simulink subsystem "rss_StrtUpRefTqCalcNeed"  (R2023a)
settings: Solver=VariableStepAuto  StartTime=0.0  StopTime=10.0  RelTol=1e-3
undefined symbols (not defined in the file): Cdbl_facStrtUpTqRiseRateMaxVal, Cdbl_nElecAgSpdMaxVal, Cdbl_tiSlwTaskSmpTi, Cdbl_trqTqMaxVal, ENM_MOTO_STATUS, ENM_STRTUP_TRQ_STATUS, Gs16_facStrtUpTqRiseRate_C, Gs16_trqMaxStrtUpTq_C
libraries: simulink x3, lib_conversion x1, lib_discrete_time_integrator x1, vhit_control_library x1
settings Model: Creator=xiaoqiang.yuan  LastModifiedBy=xiaoqiang.yuan

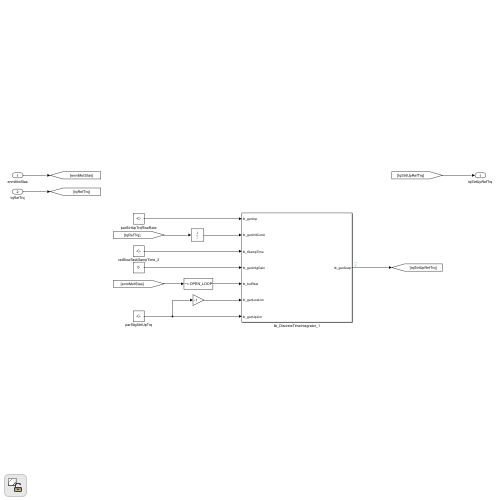
[thumbnail: Simulink's stored preview of the top-level diagram]
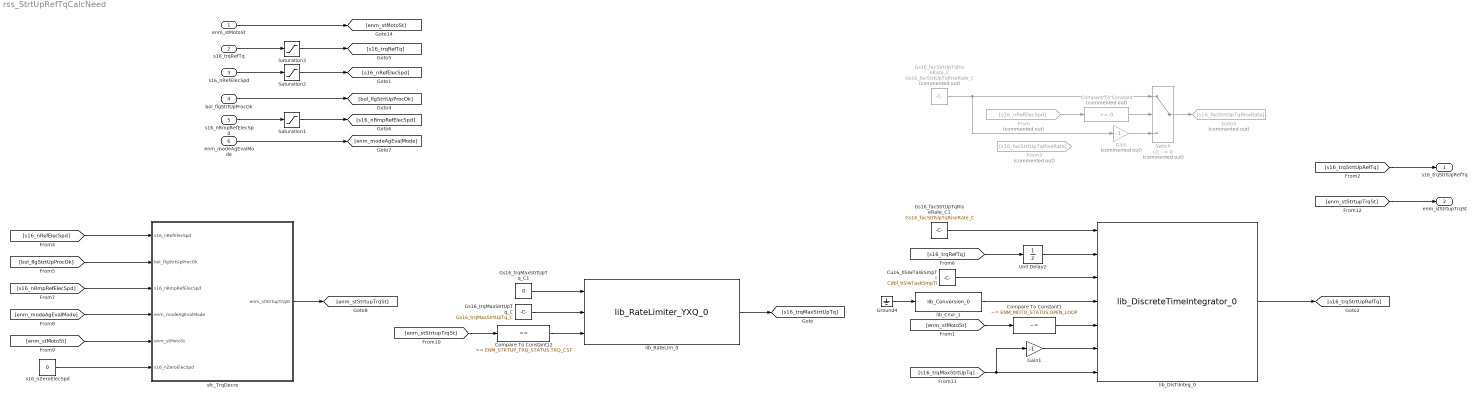
== system rss_StrtUpRefTqCalcNeed ==
  enm_stMotoSt : Inport  OutDataTypeStr=Enum: ENM_MOTO_STATUS
  s16_trqRefTq : Inport  Port=2  OutDataTypeStr=dt_Standardize_s16p15b0
  s16_nRefElecSpd : Inport  Port=3  OutDataTypeStr=dt_Standardize_s16p15b0
  bol_flgStrtUpProcOk : Inport  Port=4  OutDataTypeStr=boolean
  s16_nRmpRefElecSpd : Inport  Port=5  OutDataTypeStr=dt_Standardize_s16p15b0
  enm_modeAgEvalMode : Inport  Port=6  OutDataTypeStr=Enum: ENM_AG_POS_EVAL_MODE
  Compare To Constant : simulink/Logic and Bit Operations/Compare To Constant  Commented=on  relop=>=  const=0  OutDataTypeStr=boolean
  Compare To Constant1 : simulink/Logic and Bit Operations/Compare To Constant  relop=~=  const=ENM_MOTO_STATUS.OPEN_LOOP  OutDataTypeStr=boolean
  Compare To Constant12 : simulink/Logic and Bit Operations/Compare To Constant  relop===  const=ENM_STRTUP_TRQ_STATUS.TRQ_CST  OutDataTypeStr=boolean
  Cu16_tiSlwTaskSmpTi : Constant  Value=Cdbl_tiSlwTaskSmpTi
  From : From  Commented=on  GotoTag=s16_nRefElecSpd
  From3 : From  Commented=on  GotoTag=s16_facStrtUpTqRiseRate
  Gain : Gain  Commented=on  Gain=-1  OutDataTypeStr=Inherit: Same as input
  Gain1 : Gain  Gain=-1  OutDataTypeStr=Inherit: Inherit via back propagation
  Goto3 : Goto  Commented=on  GotoTag=s16_facStrtUpTqRiseRate
  Ground4 : Ground
  Gs16_facStrtUpTqRiseRate_C : Constant  Commented=on  Value=Gs16_facStrtUpTqRiseRate_C  OutDataTypeStr=fixdt(1,16,2^-2,0)
  Gs16_facStrtUpTqRiseRate_C1 : Constant  Value=Gs16_facStrtUpTqRiseRate_C  OutDataTypeStr=fixdt(1,16,2^-2,0)
  Gs16_trqMaxStrtUpTq_C : Constant  Value=Gs16_trqMaxStrtUpTq_C
  Gs16_trqMaxStrtUpTq_C1 : Constant  Value=0  OutDataTypeStr=dt_Standardize_s16p15b0
  Saturation1 : Saturate  UpperLimit=Cdbl_nElecAgSpdMaxVal  LowerLimit=-Cdbl_nElecAgSpdMaxVal
  Saturation2 : Saturate  UpperLimit=Cdbl_nElecAgSpdMaxVal  LowerLimit=-Cdbl_nElecAgSpdMaxVal
  Saturation3 : Saturate  UpperLimit=Cdbl_trqTqMaxVal  LowerLimit=-Cdbl_trqTqMaxVal
  Switch : Switch  Commented=on  Criteria=u2 ~= 0  SaturateOnIntegerOverflow=off  InputSameDT=off
  Unit Delay2 : UnitDelay  SampleTime=-1  HasFrameUpgradeWarning=on
  lib_Cnvr_1 : lib_conversion/lib_Conversion_0  lb_parDataType=uint8  lb_parOutpMaxVal=[]  lb_parOutpMinVal=[]  lb_parSatFlag=off
  lib_DisTiInteg_0 : lib_discrete_time_integrator/lib_DiscreteTimeIntegrator_0  lb_parMaxInpVal=Cdbl_facStrtUpTqRiseRateMaxVal  lb_parMinInpVal=-Cdbl_facStrtUpTqRiseRateMaxVal  lb_parMaxSampTime=double(Cdbl_tiSlwTaskSmpTi)  lb_parMaxIntgGain=0  lb_parAccmDataTypeMode=Same of output  lb_parOutpDataType=dt_Standardize_s16p15b0  lb_parIntgScopMode=Generic signal  lb_parSatFlag=on
  lib_RateLim_0 : vhit_control_library/lib_RateLimiter_YXQ_0  lb_parSampTime=Cdbl_tiSlwTaskSmpTi  lb_parRiseSlewRate=Gs16_facStrtUpTrqDecRiseRate_C  lb_parFallSlewRate=Gs16_facStrtUpTrqDecFallRate_C  lb_parMaxInpVal=Cdbl_trqTqMaxVal  lb_parMinInpVal=-Cdbl_trqTqMaxVal
      settings: LibrarySourceBlock=lib_rate_limiter/lib_RateLimiter_0
  s16_nZeroElecSpd : Constant  Value=0  OutDataTypeStr=dt_Standardize_s16p15b0
  sfc_TrqDecre : Stateflow chart  TreatAsAtomicUnit=on
  s16_trqStrtUpRefTq : Outport  OutDataTypeStr=dt_Standardize_s16p15b0
  enm_stStrtupTrqSt : Outport  Port=2  OutDataTypeStr=Enum: ENM_STRTUP_TRQ_STATUS
  wires:
  Gs16_facStrtUpTqRiseRate_C1/1 -> lib_DisTiInteg_0/1
  [s16_trqStrtUpRefTq] -> s16_trqStrtUpRefTq/1
  lib_Cnvr_1/1 -> lib_DisTiInteg_0/4
  [s16_trqMaxStrtUpTq] -> lib_DisTiInteg_0/7, Gain1/1
  Cu16_tiSlwTaskSmpTi/1 -> lib_DisTiInteg_0/3
  Gain1/1 -> lib_DisTiInteg_0/6
  Compare To Constant1/1 -> lib_DisTiInteg_0/5
  [enm_stMotoSt] -> Compare To Constant1/1
  lib_DisTiInteg_0/1 -> [s16_trqStrtUpRefTq]
  s16_trqRefTq/1 -> Saturation3/1
  [s16_trqRefTq] -> Unit Delay2/1
  Unit Delay2/1 -> lib_DisTiInteg_0/2
  enm_stMotoSt/1 -> [enm_stMotoSt]
  Saturation3/1 -> [s16_trqRefTq]
  Ground4/1 -> lib_Cnvr_1/1
  Saturation2/1 -> [s16_nRefElecSpd]
  s16_nRefElecSpd/1 -> Saturation2/1
  From/1 -> Compare To Constant/1
  Compare To Constant/1 -> Switch/2
  Switch/1 -> Goto3/1
  Gs16_facStrtUpTqRiseRate_C/1 -> Gain/1, Switch/1
  Gain/1 -> Switch/3
  bol_flgStrtUpProcOk/1 -> [bol_flgStrtUpProcOk]
  enm_modeAgEvalMode/1 -> [enm_modeAgEvalMode]
  Saturation1/1 -> [s16_nRmpRefElecSpd]
  s16_nRmpRefElecSpd/1 -> Saturation1/1
  s16_nZeroElecSpd/1 -> sfc_TrqDecre/6(s16_nZeroElecSpd)
  [enm_stMotoSt] -> sfc_TrqDecre/5(enm_stMotoSt)
  [enm_modeAgEvalMode] -> sfc_TrqDecre/4(enm_modeAgEvalMode)
  [s16_nRmpRefElecSpd] -> sfc_TrqDecre/3(s16_nRmpRefElecSpd)
  [bol_flgStrtUpProcOk] -> sfc_TrqDecre/2(bol_flgStrtUpProcOk)
  [s16_nRefElecSpd] -> sfc_TrqDecre/1(s16_nRefElecSpd)
  Compare To Constant12/1 -> lib_RateLim_0/3
  sfc_TrqDecre/1(enm_stStrtupTrqSt) -> [enm_stStrtupTrqSt]
  [enm_stStrtupTrqSt] -> Compare To Constant12/1
  Gs16_trqMaxStrtUpTq_C/1 -> lib_RateLim_0/2
  Gs16_trqMaxStrtUpTq_C1/1 -> lib_RateLim_0/1
  lib_RateLim_0/1 -> [s16_trqMaxStrtUpTq]
  [enm_stStrtupTrqSt] -> enm_stStrtupTrqSt/1

== stateflow chart rss_StrtUpRefTqCalcNeed/sfc_TrqDecre ==
  state TRQ_CST
    en:
    enm_stStrtupTrqSt = ENM_STRTUP_TRQ_STATUS.TRQ_CST;
  state TRQ_DECRE
    en:
    enm_stStrtupTrqSt = ENM_STRTUP_TRQ_STATUS.TRQ_DECRE;
  (default) -> TRQ_CST
  TRQ_CST -> TRQ_DECRE : [((s16_nRefElecSpd ~= s16_nZeroElecSpd && bol_flgStrtUpProcOk && abs(s16_nRmpRefElecSpd) >= abs(Gs16_nMinSenlRefElecSpd_C)) || ...
      | enm_modeAgEvalMode ~= ENM_AG_POS_EVAL_MODE.SENSORLESS) && enm_stMotoSt == ENM_MOTO_STATUS.OPEN_LOOP]
  TRQ_DECRE -> TRQ_CST : [enm_stMotoSt ~= ENM_MOTO_STATUS.OPEN_LOOP]
  data: s16_nRefElecSpd input dt_Standardize_s16p15b0; bol_flgStrtUpProcOk input boolean; s16_nRmpRefElecSpd input dt_Standardize_s16p15b0; enm_modeAgEvalMode input Enum: ENM_AG_POS_EVAL_MODE; Gs16_nMinSenlRefElecSpd_C parameter; enm_stMotoSt input Enum: ENM_MOTO_STATUS; enm_stStrtupTrqSt output Enum: ENM_STRTUP_TRQ_STATUS; s16_nZeroElecSpd input dt_Standardize_s16p15b0
